simulink model "dc_to_mod2"  (Simulink 8.1)
settings: Solver=ode3  StartTime=0.0  StopTime=80e-3  RelTol=1e-3
undefined symbols (not defined in the file): Fs, input_dc, modctrl, OSR
libraries: dspsigops x3, dsparch4 x1, dspsrcs4 x1
settings Model: Creator=amyles  LastModifiedBy=amyles
settings DataIOCC: MaxDataPoints=50000
settings DebuggingCC: StrictBusMsg=Warning

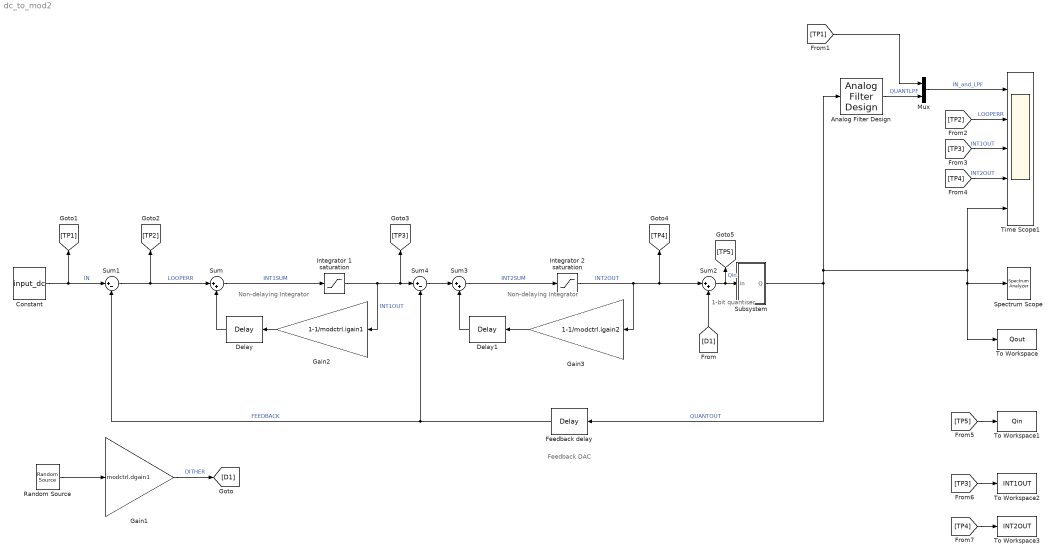
== system dc_to_mod2 ==
  note: 1-bit quantiser
  note: Non-delaying Integrator
  note: Feedback DAC
  note: Non-delaying Integrator
  Analog Filter Design : dsparch4/Analog Filter Design  method=Bessel  filttype=Lowpass  N=8  Wlo=pi*Fs/OSR  Whi=80  Rp=2  Rs=40
  Constant : Constant  Value=input_dc  SampleTime=1/Fs
  Delay : dspsigops/Delay  InputProcessing=Inherited (this choice will be removed - see release notes)  dly_unit=Samples  delay=1  ic_detail=off  dif_ic_for_ch=off  dif_ic_for_dly=off  ic=0  reset_popup=None
  Delay1 : dspsigops/Delay  InputProcessing=Inherited (this choice will be removed - see release notes)  dly_unit=Samples  delay=1  ic_detail=off  dif_ic_for_ch=off  dif_ic_for_dly=off  ic=0  reset_popup=None
  Feedback delay : dspsigops/Delay  InputProcessing=Inherited (this choice will be removed - see release notes)  dly_unit=Samples  delay=1  ic_detail=off  dif_ic_for_ch=off  dif_ic_for_dly=off  ic=0  reset_popup=None
  Gain1 : Gain  Gain=modctrl.dgain1
      settings: AttributesFormatString=Dither level adjust
  Gain2 : Gain  Gain=1-1/modctrl.igain1
      settings: AttributesFormatString=Integrator leakage
  Gain3 : Gain  Gain=1-1/modctrl.igain2
      settings: AttributesFormatString=Integrator leakage
  Integrator 1 saturation : Saturate  UpperLimit=modctrl.isat1  LowerLimit=-(modctrl.isat1)
  Integrator 2 saturation : Saturate  UpperLimit=modctrl.isat2  LowerLimit=-(modctrl.isat2)
  Mux : Mux  Inputs=2
  Random Source : dspsrcs4/Random Source  SrcType=Uniform  NormMethod=Ziggurat  CltLength=12  MinVal=-1  MaxVal=1  MeanVal=0  VarVal=1  RepMode=Not repeatable  rawSeed=1  IsInherit=off  SampMode=Discrete  SampTime=1/Fs  SampFrame=1  DataType=Double  OutComplex=Real
      settings: AttributesFormatString=Dither source
  Spectrum Scope : SpectrumAnalyzer
      settings: CopyFcn=scopeextensions.ScopeBlock.callback(gcbh, 'onBlockCopy', gcbh);  DeleteFcn=scopeextensions.ScopeBlock.callback(gcbh, 'onBlockDelete');  PreSaveFcn=scopeextensions.ScopeBlock.callback(gcbh, 'onModelSave');  NameChangeFcn=scopeextensions.ScopeBlock.callback(gcbh, 'onBlockRename');  CloseFcn=scopeextensions.ScopeBlock.callback(gcbh, 'onBlockClose');  PreDeleteFcn=scopeextensions.ScopeBlock.callback(gcbh, 'onBlockPreDelete');
  Subsystem : Subsystem
      settings: AttributesFormatString=1-bit quantiser
  Sum : Sum  Inputs=|++
      settings: AttributesFormatString=Integrator summer
  Sum1 : Sum  Inputs=|+-
      settings: AttributesFormatString=Modulator input\nloop servo error (input - fbk)
  Sum2 : Sum  Inputs=|++
  Sum3 : Sum  Inputs=|++
      settings: AttributesFormatString=Integrator summer
  Sum4 : Sum  Inputs=|+-
  Time Scope1 : Scope  NumInputPorts=5
      settings: TimeRange=0.08  YMin=-5~-1.2~-2.5~-1.2~-5  YMax=5~1.2~2.5~1.2~5  DataFormat=Structure  MaxDataPoints=80000
  To Workspace : ToWorkspace  VariableName=Qout  SampleTime=-1
      settings: AttributesFormatString=Export SDM output\nto workspace for\npost-processing
  To Workspace1 : ToWorkspace  VariableName=Qin  SampleTime=-1
      settings: AttributesFormatString=Export SDM output\nto workspace for\npost-processing
  To Workspace2 : ToWorkspace  VariableName=INT1OUT  SampleTime=-1
  To Workspace3 : ToWorkspace  VariableName=INT2OUT  SampleTime=-1
  wires:
  Delay/1 -> Sum/2
  Sum/1 -> Integrator 1 saturation/1  "INT1SUM"
  Sum1/1 -> Sum/1, [TP2]  "LOOPERR"
  Feedback delay/1 -> Sum1/2, Sum4/2  "FEEDBACK"
  Constant/1 -> Sum1/1, [TP1]  "IN"
  Analog Filter Design/1 -> Mux/2  "QUANTLPF"
  Sum2/1 -> Subsystem/1(in), [TP5]  "Qin"
  Gain2/1 -> Delay/1
  Subsystem/1(Q) -> Analog Filter Design/1, To Workspace/1, Spectrum Scope/1, Time Scope1/5, Feedback delay/1  "QUANTOUT"
  Mux/1 -> Time Scope1/1  "IN_and_LPF"
  Delay1/1 -> Sum3/2
  Sum3/1 -> Integrator 2 saturation/1  "INT2SUM"
  Sum4/1 -> Sum3/1
  Gain3/1 -> Delay1/1
  Integrator 2 saturation/1 -> Gain3/1, Sum2/1, [TP4]  "INT2OUT"
  Integrator 1 saturation/1 -> Gain2/1, Sum4/1, [TP3]  "INT1OUT"
  Random Source/1 -> Gain1/1
  Gain1/1 -> [D1]  "DITHER"
  [D1] -> Sum2/2
  [TP1] -> Mux/1
  [TP2] -> Time Scope1/2  "LOOPERR"
  [TP3] -> Time Scope1/3  "INT1OUT"
  [TP4] -> Time Scope1/4  "INT2OUT"
  [TP5] -> To Workspace1/1
  [TP3] -> To Workspace2/1
  [TP4] -> To Workspace3/1

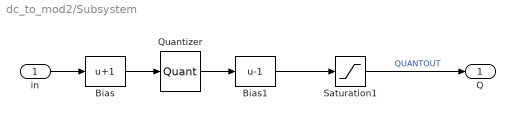
== system dc_to_mod2/Subsystem ==
  in : Inport
  Bias : Bias  Bias=1
      settings: AttributesFormatString=Need offset to give\nMID-RISE quantiser
  Bias1 : Bias  Bias=-1
  Quantizer : Quantizer  QuantizationInterval=2  LinearizeAsGain=off
  Saturation1 : Saturate  UpperLimit=1  LowerLimit=-1
      settings: AttributesFormatString=Limit quantiser\noutput to +/-1
  Q : Outport
  wires:
  Bias/1 -> Quantizer/1
  Quantizer/1 -> Bias1/1
  Bias1/1 -> Saturation1/1
  in/1 -> Bias/1
  Saturation1/1 -> Q/1  "QUANTOUT"
